simulink model "Lab1_Simulink"  (R2023b)
settings: Solver=VariableStepAuto  StartTime=0.0  StopTime=20.0  RelTol=1e-3
settings Model: Creator=2361266  LastModifiedBy=htetaung

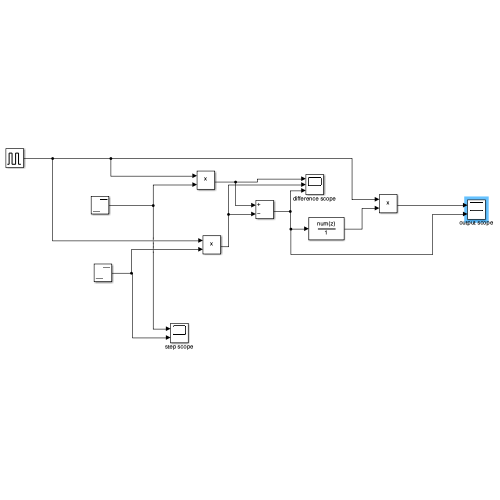
[thumbnail: Simulink's stored preview of the top-level diagram]
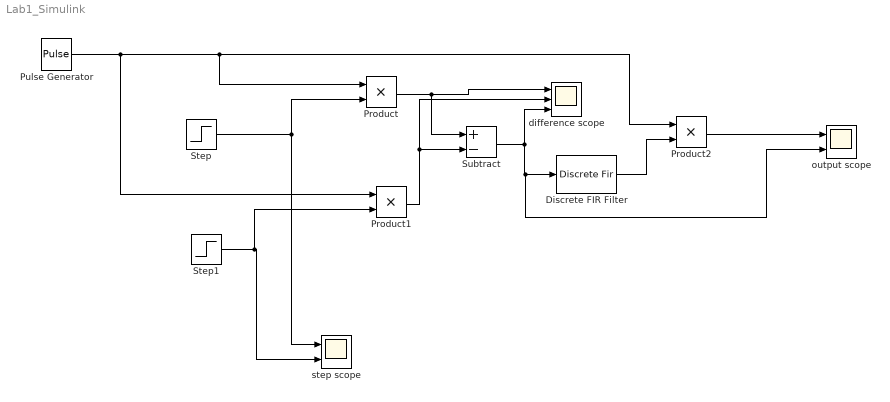
== system Lab1_Simulink ==
  Discrete FIR Filter : DiscreteFir  Coefficients=[1,1,1,1]  SampleTime=1
  Product : Product
  Product1 : Product
  Product2 : Product
  Pulse Generator : DiscretePulseGenerator  PulseType=Time based  Period=1  PulseWidth=5
  Step : Step  Time=4  SampleTime=0
  Step1 : Step  Time=0  SampleTime=0
  Subtract : Sum  Inputs=+-
  difference scope : Scope  NumInputPorts=3
  output scope : Scope  NumInputPorts=2
  step scope : Scope  NumInputPorts=2
  wires:
  Product/1 -> Subtract/1, difference scope/1
  Pulse Generator/1 -> Product1/1, Product2/1, Product/1
  Step/1 -> Product/2, step scope/1
  Product1/1 -> Subtract/2, difference scope/2
  Subtract/1 -> difference scope/3, output scope/2, Discrete FIR Filter/1
  Discrete FIR Filter/1 -> Product2/2
  Product2/1 -> output scope/1
  Step1/1 -> Product1/2, step scope/2
